simulink library "csu_ecl_egc_command_latch_lib"  (R2014b)
settings: Solver=ode45  StartTime=0.0  StopTime=10.0  RelTol=1e-3
values from neighbouring files (symbols this model uses):
  egc_msgid = fsw_commands('egc_reset_ctrs').msgid    [csu_ecl_egc_command_latch_init.m]
libraries: simulink x5, util_event_lib x3, util_info_lib x1
settings Model: Creator=mstewart  LastModifiedBy=mstewart

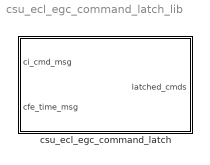
== system csu_ecl_egc_command_latch_lib ==
  csu_ecl_egc_command_latch : Subsystem

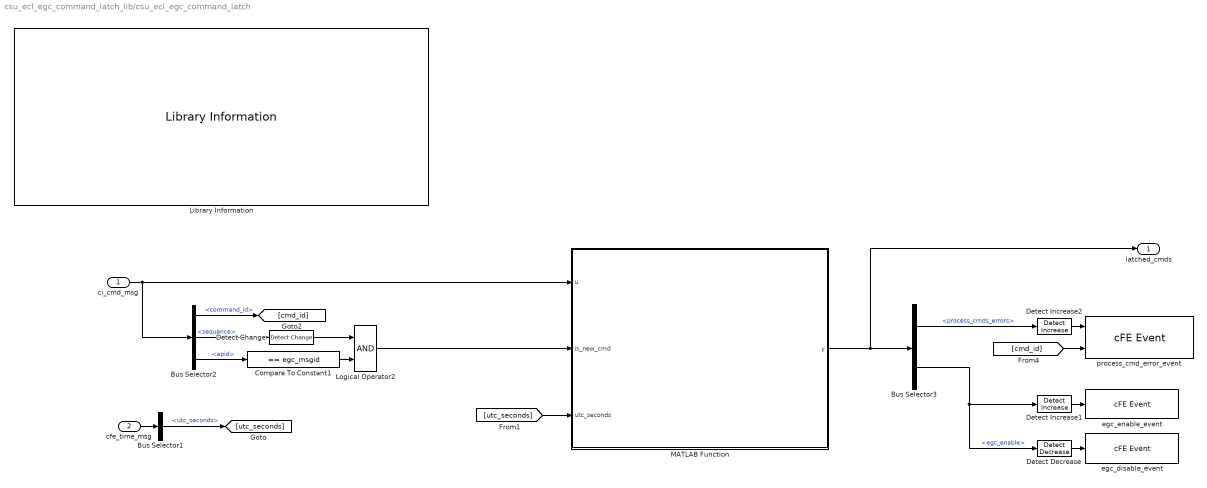
== system csu_ecl_egc_command_latch_lib/csu_ecl_egc_command_latch ==
  ci_cmd_msg : Inport  OutDataTypeStr=Bus: ci_cmd_msg
  cfe_time_msg : Inport  Port=2  OutDataTypeStr=Bus: cfe_time_msg
  Bus Selector1 : BusSelector  OutputSignals=utc_seconds
  Bus Selector2 : BusSelector  OutputSignals=command_id,sequence,apid
  Bus Selector3 : BusSelector  OutputSignals=process_cmds_errors,egc_enable
  Compare To Constant1 : simulink/Logic and Bit Operations/Compare To Constant  relop===  const=egc_msgid  OutDataTypeStr=boolean
  Detect Change : simulink/Logic and Bit Operations/Detect Change  vinit=0  InputProcessing=Inherited  OutDataTypeStr=boolean
  Detect Decrease : simulink/Logic and Bit Operations/Detect Decrease  vinit=0.0  InputProcessing=Inherited  OutDataTypeStr=boolean
  Detect Increase1 : simulink/Logic and Bit Operations/Detect Increase  vinit=0.0  InputProcessing=Inherited  OutDataTypeStr=boolean
  Detect Increase2 : simulink/Logic and Bit Operations/Detect Increase  vinit=0.0  InputProcessing=Inherited  OutDataTypeStr=boolean
  Library Information : util_info_lib/Library Information  owner='NONE'
  Logical Operator2 : Logic  AllPortsSameDT=off  OutDataTypeStr=boolean
  MATLAB Function : MATLAB Function  TreatAsAtomicUnit=on
  egc_disable_event : util_event_lib/cFE Event  event_message='EGC disabled'  event_id=20  event_severity=INFORMATION  event_use_enums=off  event_enum_types={}
  egc_enable_event : util_event_lib/cFE Event  event_message='EGC enabled'  event_id=20  event_severity=INFORMATION  event_use_enums=off  event_enum_types={}
  process_cmd_error_event : util_event_lib/cFE Event  event_message='Error processing command with command code %u'  event_id=21  event_severity=ERROR  event_use_enums=off  event_enum_types={}
  latched_cmds : Outport
  wires:
  ci_cmd_msg/1 -> Bus Selector2/1, MATLAB Function/1(u)
  Detect Increase1/1 -> egc_enable_event/1
  cfe_time_msg/1 -> Bus Selector1/1
  Bus Selector1/1 -> [utc_seconds]  "<utc_seconds>"
  Bus Selector2/1 -> [cmd_id]  "<command_id>"
  Bus Selector2/2 -> Detect Change/1  "<sequence>"
  [utc_seconds] -> MATLAB Function/3(utc_seconds)
  Logical Operator2/1 -> MATLAB Function/2(is_new_cmd)
  [cmd_id] -> process_cmd_error_event/2
  Detect Increase2/1 -> process_cmd_error_event/1
  Bus Selector2/3 -> Compare To Constant1/1  "<apid>"
  Detect Change/1 -> Logical Operator2/1
  Compare To Constant1/1 -> Logical Operator2/2
  Bus Selector3/1 -> Detect Increase2/1  "<process_cmds_errors>"
  Bus Selector3/2 -> Detect Decrease/1, Detect Increase1/1  "<egc_enable>"
  Detect Decrease/1 -> egc_disable_event/1
  MATLAB Function/1(y) -> latched_cmds/1, Bus Selector3/1

== matlab function csu_ecl_egc_command_latch_lib/csu_ecl_egc_command_latch/MATLAB Function ==
  data: u input Bus: ci_cmd_msg; y output Bus: ecl_bus_msg; is_new_cmd input boolean; utc_seconds input uint32; ecl_cmd_indices parameter
function y = decode_and_latch(u, is_new_cmd, utc_seconds, ecl_cmd_indices)
%#codegen

persistent latched_values;

if isempty(latched_values)
    latched_values.cfe_tlm_header_align = zeros(4,1,'uint8');
    latched_values.process_cmds_counter = uint16(0);
    latched_values.process_cmds_errors = uint16(0);
    latched_values.egc_enable = uint8(0);
end

if is_new_cmd

    if (u.command_id == ecl_cmd_indices.egc_reset_ctrs)
        latched_values.process_cmds_counter = uint16(0);
        latched_values.process_cmds_errors = uint16(0);
        
    elseif (u.command_id == ecl_cmd_indices.egc_enable)
        latched_values.egc_enable = uint8(1);
        latched_values.process_cmds_counter = latched_values.process_cmds_counter + 1;
        
    elseif (u.command_id == ecl_cmd_indices.egc_disable)
        latched_values.egc_enable = uint8(0);
        latched_values.process_cmds_counter = latched_values.process_cmds_counter + 1;
    
    else
        latched_values.process_cmds_errors = latched_values.process_cmds_errors + 1;
    end
    
end

y = latched_values;
